simulink model "ConfiguredVirtualVehicleModel"  (R2025b)
settings: Solver=daessc  StartTime=0  StopTime=2474  FixedStep=.001  RelTol=1e-2  EnableMultiTasking=on
StopFcn:
  | %toc
undefined symbols (not defined in the file or in its folder): AccelOvrCmd, CtrlTcuInitGear, DecelOvrCmd, Disabled, DriverPreviewDist, EnblAccelOvr, EnblDecelCmd, EnblSteerCmd, EnvAbsPrs, EnvAirTemp, EnvGrvty, EnvNomFrictionScaling, EnvNominalGrade, EnvWindVelX, EnvWindVelY, EnvWindVelZ, FTP75, MotoFrmInert, MotoFrmLngth, MotoFrmMass, MotoLowrFrntFrkMass, MotoRearArmLngth, MotoRearArmMass, MotoUpprFrntFrkMass, RiderLkAhdPtDstGain, RiderMass, ScnAccTbl, ScnBrkTbl, ScnCRMaxLatAccel, ScnCRRadius, ScnDLCGateLongPos, ScnDLCLatRef, ScnDLCLatRefOffset, ScnDLCLongRefBpt, ScnDLCLongRefStartPos, ScnDLCVehicleWidth, ScnFHCounterDwellTime, ScnFHInitialDwellTime, ScnFHReturnTime, ScnFHRollRateZeroCross, ScnFHSteerAmp, ScnFHSteerSpeed, ScnISHandwheelRate, ScnISMaxHandwheelAng, ScnISMaxLatAccel, ScnISSteerHoldTime, ScnLongPosBpts, ScnLongVelRef, ScnOvalTrackl, ScnOvalTrackpdst, ScnOvalTrackr, ScnSDDwellTime, ScnSDSteerAmp, ScnSDSteerFreq, ScnSSFinalFreq, ScnSSSteerAmp, ScnSSSweepTime, ScnStartTime, ScnStrgAngTbl, ScnStrgTrqTbl ... (+10)
libraries: simulink x16, vehdynlibscenariocommon x9, sm_lib x6, autolibshared x4, nesl_utility x4, vehdynlibviscommon x3, sim3dgroundtruthsensorlib x2, vehdynlibdriver x2, sharedtransform x1, autolibutils x1, sim3dautolib x1, sim3dlib x1
(part 1 of 6)
settings Model: DataDictionary=VirtualMotoTemplate.sldd  ModifiedByFormat=The MathWorks, Inc.  SimulationMode=accelerator  PauseTimes=23.4  PacingRate=0.001000  Creator=The MathWorks, Inc.  LastModifiedBy=The MathWorks, Inc.
settings SolverCC: DaesscMode=Fast  ZeroCrossAlgorithm=Adaptive  AlgebraicLoopSolver=TrustRegion  AutoInsertRateTranBlk=on  InsertRTBMode=Never (minimum delay)  DecoupledContinuousIntegration=on  MinimalZcImpactIntegration=on  MaxZcPerStep=1.0
settings DataIOCC: DSMLogging=off  ReturnWorkspaceOutputs=off
settings OptimizationCC: ReuseModelBlockBuffer=off
settings DebuggingCC: SignalInfNanChecking=error  ArtificialAlgebraicLoopMsg=none  MaskedZcDiagnostic=none  IgnoredZcDiagnostic=none  UnconnectedInputMsg=warning  UnconnectedOutputMsg=warning  UnconnectedLineMsg=warning  PregeneratedLibrarySubsystemCodeDiagnostic=none  SubsystemReferenceDiagnosticForUnitTest=warning  ArithmeticOperatorsInVariantConditions=warning
settings HardwareCC: UseEmbeddedCoderFeatures=off
settings ModelReferenceCC: EnableRefExpFcnMdlSchedulingChecks=on  ModelReferenceMinAlgLoopOccurrences=on  PropagateSignalLabelsOutOfModel=off
settings SFSimCC: SimUseLocalCustomCode=off
settings RTWCC: RTWUseLocalCustomCode=off  GPUComputeCapability=3.5  DLArmComputeVersion=19.05  LargeConstantGeneration=WriteOnlyDNNConstantsToDataFiles
settings ExplorerConfigSet: SimMechanicsOpenEditorOnUpdate=off  InternalSimMechanicsExplorerSettings="<ExplorerConfiguration><canonicalview>default</canonicalview><AnimationSetting><BasePlaybackSpeed>1.0</BasePlaybackSpeed><PlaybackSpeedFactor>0.5</PlaybackSpeedFactor></AnimationSetting><TilePanel><TileInfo><Tiles Columns=\"1\" Count=\"1\" Rows=\"1\"><Column Weight=\"1\"/><Row Weight=\"1\"/><Tile Height=\"1\" Width=\"1\" X=\"0\" Y=\"0\"/></Tiles></TileInfo><SceneInfo><SceneViewer><BGColor><R>0.60000002384185791</R><G>0.60000002384185791</G><B>0.60000002384185791</B></BGColor><Camera><DoPerspective>on</DoPerspective><Position><X>48.3730560002180638</X><Y>0.69720714407681017</Y><Z>1.00624025938607131</Z></Position><Center><X>47.6181790802191784</X><Y>1.35307362107727269</Y><Z>1.00624025938607131</Z></Center><Up><X>0</X><Y>0</Y><Z>1</Z></Up><ViewLimDist>1</ViewLimDist><YLim>0.466307658154998583</YLim><XLim>1.00155607891196818</XLim></Camera></SceneViewer></SceneInfo></TilePanel><MechEditorPanel><Cameras><Camera><Id>Camera1</Id><Value><Name>InplaneRightSide</Name><NativeCamera><PositionTrackingFeature>Motorcycle_Vehicle.Body_Steer_Suspension_Wheels.Body_Steer_Suspension_Wheels.In_Plane_Model.Chassis_Tires_and_Areo.Chassis_Body_Suspension_and_Steering.CHASSIS.Chassis_body.CPRr.Camera.Right.base.R</PositionTrackingFeature><CenterTrackingFeature>Motorcycle_Vehicle.Body_Steer_Suspension_Wheels.Body_Steer_Suspension_Wheels.In_Plane_Model.Chassis_Tires_and_Areo.Chassis_Body_Suspension_and_Steering.CHASSIS.Chassis_body.CPRr.Camera.Right.target.R</CenterTrackingFeature><UpVectorTrackingFeature>Motorcycle_Vehicle.Body_Steer_Suspension_Wheels.Body_Steer_Suspension_Wheels.In_Plane_Model.Chassis_Tires_and_Areo.Chassis_Body_Suspension_and_Steering.CHASSIS.Chassis_body.CPRr.Camera.Right.target.R</UpVectorTrackingFeature><CenterTrackingOrigin>off</CenterTrackingOrigin><CenterTrackingDirection>-Y</CenterTrackingDirection><UpVectorTrackingDirection>-Z</UpVectorTrackingDirection></NativeCamera></Value></Camera><Camera><Id>Camera2</Id><Value><Name>OutofPlaneRightSide</Name><NativeCamera><PositionTrackingFeature>Motorcycle_Vehicle.Body_Steer_Suspension_Wheels.Body_Steer_Suspension_Wheels.Out_of_Plane_Model.Chassis_Tires_and_Areo.Chassis_Body_Suspension_and_Steering.CHASSIS.Chassis_body.CPRr.Camera.Right.base.R</PositionTrackingFeature><CenterTrackingFeature>Motorcycle_Vehicle.Body_Steer_Suspension_Wheels.Body_Steer_Suspension_Wheels.Out_of_Plane_Model.Chassis_Tires_and_Areo.Chassis_Body_Suspension_and_Steering.CHASSIS.Chassis_body.CPRr.Camera.Right.base.R</CenterTrackingFeature><UpVectorTrackingFeature>Motorcycle_Vehicle.Body_Steer_Suspension_Wheels.Body_Steer_Suspension_Wheels.Out_of_Plane_Model.Chassis_Tires_and_Areo.Chassis_Body_Suspension_and_Steering.CHASSIS.Chassis_body.CPRr.Camera.Right.base.R</UpVectorTrackingFeature><CenterTrackingOrigin>off</CenterTrackingOrigin><CenterTrackingDirection>-Y</CenterTrackingDirection><UpVectorTrackingDirection>-Z</UpVectorTrackingDirection></NativeCamera></Value></Camera></Cameras><GfxPanelCameraMap><MapElement CameraMLId=\"Camera2\" GfxPanelIndex=\"0\"/></GfxPanelCameraMap><VideoCreator><PlaybackSpeedRatio>1.0</PlaybackSpeedRatio><FrameRate>30</FrameRate><VideoFormat>Motion JPEG AVI</VideoFormat><FrameSize>auto</FrameSize></VideoCreator></MechEditorPanel></ExplorerConfiguration>"

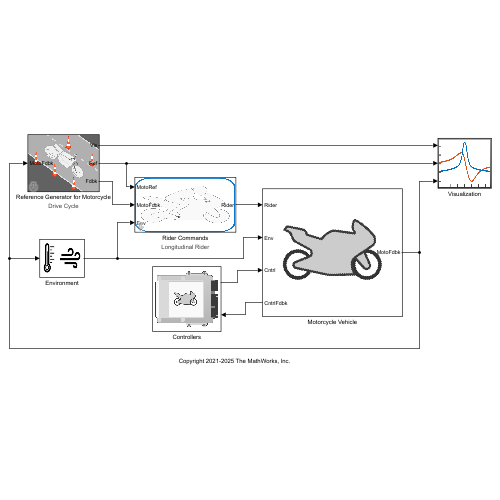
[thumbnail: Simulink's stored preview of the top-level diagram]
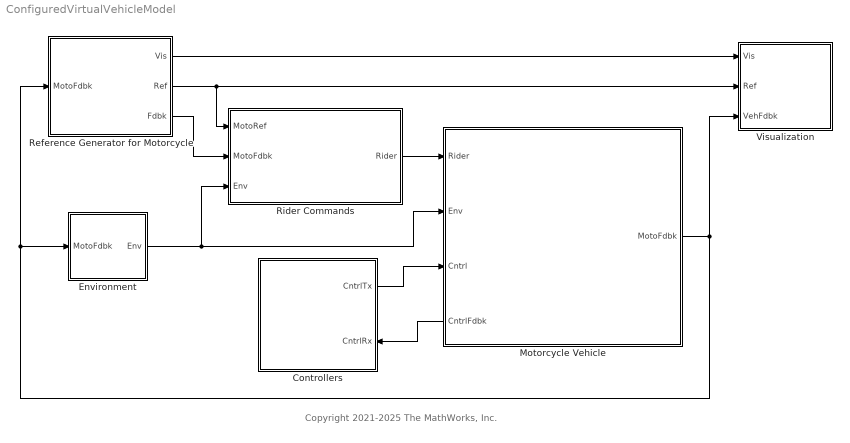
== system ConfiguredVirtualVehicleModel ==
  note: Copyright 2021-2025 The MathWorks, Inc.
  Controllers : Subsystem
      settings: PortSchema="{\"entries\":[{\"content\":{\"sides\":[{\"content\":{},\"type\":\"ConnectorPlacement.EquallySpacedRectSide\",\"uuid\":\"d3abfdf3-59f3-4762-8e4e-957745a11e2c\"},{\"content\":{\"connectorIds\":[\"Out1\",\"In1\"],\"side\":\"RIGHT\"},\"type\":\"ConnectorPlacement.EquallySpacedRectSide\",\"uuid\":\"4c115717-9c17-4631-bd95-1f831e7f83d7\"},{\"content\":{\"side\":\"TOP\"},\"type\":\"ConnectorPlacement.EquallySpacedRectSide\",\"uuid\":\"d2ccb451-5fc1-4147-9a0c-1582624fa182\"}]},\"type\":\"ConnectorPlacement.EquallySpacedConnector\",\"uuid\":\"cab9e2c1-ce8a-4f9c-a024-cef64f8d49c6\"}],\"packageUris\":[\"http://schema.mathworks.com/mf0/Connector/R2020b\"],\"version\":\"1.0\"}"
      mask Display: image('motoECU.png')
  Environment : Subsystem
      mask Display: image('Enviroment.png')
  Motorcycle Vehicle : Subsystem
      settings: PortSchema="{\"entries\":[{\"content\":{\"sides\":[{\"content\":{\"connectorIds\":[\"In1\",\"In2\",\"In3\",\"Out2\"]},\"type\":\"ConnectorPlacement.EquallySpacedRectSide\",\"uuid\":\"175d7041-2aff-4cd5-b9c0-3998d48105ea\"},{\"content\":{\"connectorIds\":[\"Out1\"],\"side\":\"RIGHT\"},\"type\":\"ConnectorPlacement.EquallySpacedRectSide\",\"uuid\":\"0f698ea4-f06f-4552-98b1-af1f0960853e\"},{\"content\":{\"side\":\"TOP\"},\"type\":\"ConnectorPlacement.EquallySpacedRectSide\",\"uuid\":\"8127d405-6a03-4548-a956-3e3bb7246319\"}]},\"type\":\"ConnectorPlacement.EquallySpacedConnector\",\"uuid\":\"b217a386-2802-4b5f-8626-423e606b91b2\"}],\"packageUris\":[\"http://schema.mathworks.com/mf0/Connector/R2020b\"],\"version\":\"1.0\"}"
      mask Display: image('moto.png')
  Reference Generator for Motorcycle : Subsystem  Priority=1  mask(Reference Generator){manType=Drive Cycle, manOverride=off, SpdCtrlOverride=off, prevType=Drive Cycle, t_start=ScnStartTime, xdot_r=ScnLongVelRef, xdotUnit=mph, steerDir=off, aMode=2, RidTrajContGl=RiderLkAhdPtDstGain, omega_hw=ScnISHandwheelRate, theta_max=ScnISMaxHandwheelAng, t_stop=ScnISSteerHoldTime, ay_max=ScnISMaxLatAccel, ay_stop=off, XGate=ScnDLCGateLongPos, xStart=ScnDLCLongRefStartPos, vehW=ScnDLCVehicleWidth, latoff=ScnDLCLatRefOffset, latRefbp=ScnDLCLongRefBpt, latRef=ScnDLCLatRef, t_sweep=ScnSSSweepTime, theta_hw=ScnSSSteerAmp, theta_hw_final=ScnSSFinalFreq, steerF=ScnSDSteerFreq, steerA=ScnSDSteerAmp, tdwell=ScnSDDwellTime, R=ScnCRRadius*0.5, cr_ay_max=ScnCRMaxLatAccel, cr_ay_stop=off, Trajl=ScnOvalTrackl, Trajr=ScnOvalTrackr, Trajpointdist=ScnOvalTrackpdst, TrajDataSource=Variable, TrajDatFileCSV=ScnUDTrackCSVFile, TrajDatFile=ScnUDTrackMATFile, CoordinateX=ScnUDTrackCoordX, CoordinateY=ScnUDTrackCoordY, steerRate=ScnFHSteerSpeed, steerAFH=ScnFHSteerAmp, pFdbk=off, tDwell1=ScnFHInitialDwellTime, tDwell2=ScnFHCounterDwellTime, tSteer3=ScnFHReturnTime, pZero=ScnFHRollRateZeroCross, cycleVar=FTP75, xdot_wot1=90, srcUnit=mph, t_wot2=ScnTimeToStrtDecel, OverrideType=Steering torque override, ActType=Time-based activation, TimeBpts=ScnTimeBpts, LongPosBpts=ScnLongPosBpts, StrgAngTbl=ScnStrgAngTbl, StrgTrqTbl=ScnStrgTrqTbl, AccTbl=ScnAccTbl, BrkTbl=ScnBrkTbl, simTime=2474, engine3D=Disabled, SceneDesc=Open surface, dt3D=.03, defaultPos=User-specified, X_o=0, Y_o=0, Z_o=0, phi_o=0, theta_o=0, psi_o=0}
      mask prompts: manType "vdynblks:vehdynManConstantRadius:blkPrm_manType"; manOverride "vdynblks:vehdynManConstantRadius:blkPrm_manOverride"; SpdCtrlOverride "Speed control override"; t_start "vdynblks:vehdynManConstantRadius:blkPrm_t_start"; xdot_r "vdynblks:vehdynManConstantRadius:blkPrm_xdot_r"; xdotUnit "Simulink:blkprm_prompts:OutputUnit_EditField"; steerDir "vdynblks:vehdynManConstantRadius:blkPrm_steerDir"; RidTrajContGl "Gain that determines the distance to the look ahead point, RidContGl [s]:"; omega_hw "vdynblks:vehdynManConstantRadius:blkPrm_omega_hw"; theta_max "vdynblks:vehdynManConstantRadius:blkPrm_theta_max"; t_stop "vdynblks:vehdynManConstantRadius:blkPrm_t_stop"; ay_max "vdynblks:vehdynManConstantRadius:blkPrm_ay_max"; ay_stop "vdynblks:vehdynManConstantRadius:blkPrm_ay_stop"; XGate "vdynblks:vehdynManConstantRadius:blkPrm_XGate"; xStart "vdynblks:vehdynManConstantRadius:blkPrm_xStart"; vehW "vdynblks:vehdynManConstantRadius:blkPrm_vehW"; latoff "vdynblks:vehdynManConstantRadius:blkPrm_latoff"; latRefbp "vdynblks:vehdynManConstantRadius:blkPrm_latRefbp"; latRef "vdynblks:vehdynManConstantRadius:blkPrm_latRef"; t_sweep "vdynblks:vehdynManConstantRadius:blkPrm_t_sweep"; theta_hw "vdynblks:vehdynManConstantRadius:blkPrm_theta_hw"; theta_hw_final "vdynblks:vehdynManConstantRadius:blkPrm_theta_hw_final"; steerF "vdynblks:vehdynManConstantRadius:blkPrm_steerF"; steerA "vdynblks:vehdynManConstantRadius:blkPrm_steerA"; tdwell "vdynblks:vehdynManConstantRadius:blkPrm_tdwell"; R "vdynblks:vehdynManConstantRadius:blkPrm_R"; cr_ay_max "vdynblks:vehdynManConstantRadius:blkPrm_cr_ay_max"; cr_ay_stop "vdynblks:vehdynManConstantRadius:blkPrm_cr_ay_stop"; Trajl "vdynblks:vehdynManOvalTrack:blkDlg_OTStLen"; Trajr "vdynblks:vehdynManOvalTrack:blkDlg_OTTRad"; Trajpointdist "vdynblks:vehdynManOvalTrack:blkDlg_OTCIntvl"; TrajDataSource "vdynblks:vehdynManUserDefinedTrack:blkDlg_DatSrcGroup"; TrajDatFileCSV "vdynblks:vehdynManUserDefinedTrack:blkDlg_TrkDatFile"; TrajDatFile "vdynblks:vehdynManUserDefinedTrack:blkDlg_TrkDatFile"; CoordinateX "vdynblks:vehdynManUserDefinedTrack:blkDlg_UDTVarX"; CoordinateY "vdynblks:vehdynManUserDefinedTrack:blkDlg_UDTVarY"; steerRate "vdynblks:vehdynManFishook:blkPrm_steerRate"; steerAFH "vdynblks:vehdynManConstantRadius:blkPrm_steerAFH"; pFdbk "vdynblks:vehdynManFishook:blkPrm_pFdbk"; tDwell1 "vdynblks:vehdynManFishook:blkPrm_tDwell1"; tDwell2 "vdynblks:vehdynManFishook:blkPrm_tDwell2"; tSteer3 "vdynblks:vehdynManFishook:blkPrm_tSteer3"; pZero "vdynblks:vehdynManFishook:blkPrm_pZero"; cycleVar "autoblks_shared:autoblkDriveCycleSource:blkPrm_cycleVar"; xdot_wot1 "autoblks_shared:autoblkDriveCycleSource:blkPrm_xdot_wot1"; srcUnit "autoblks_shared:autoblkDriveCycleSource:blkPrm_srcUnit"; t_wot2 "autoblks_shared:autoblkDriveCycleSource:blkPrm_t_wot2"; OverrideType "Override type:"; ActType "Test activation type:"; TimeBpts "Time breakpoints, TimeBpts [t]:"; LongPosBpts "Longitudinal position breakpoints, LongPosBpts [m]:"; StrgAngTbl "Steering angle table, StrgAngTbl [rad]:"; StrgTrqTbl "Steering torque table, StrgTrqTbl [N*m]:"; AccTbl "Acceleration table, AccTbl [-]:"; BrkTbl "Brake table, BrkTbl [-]:"; simTime "vdynblks:vehdynManConstantRadius:blkPrm_simTime"; engine3D "vdynblks:vehdynManConstantRadius:blkPrm_engine3D"; SceneDesc "vdynblks:vehdynManConstantRadius:blkPrm_SceneDesc"; dt3D "vdynblks:vehdynManConstantRadius:blkPrm_dt3D"; X_o "vdynblks:vehdynManConstantRadius:blkPrm_X_o"; Y_o "vdynblks:vehdynManConstantRadius:blkPrm_Y_o"; Z_o "vdynblks:vehdynManConstantRadius:blkPrm_Z_o"; phi_o "vdynblks:vehdynManConstantRadius:blkPrm_phi_o"; theta_o "vdynblks:vehdynManConstantRadius:blkPrm_theta_o"; psi_o "vdynblks:vehdynManConstantRadius:blkPrm_psi_o"
      mask help: vdynblks:vehdynManConstantRadius:blkDesc
      mask init:
      | [~]=vdynblksrefconfig(gcb,0);
      settings: AttributesFormatString=%<manType>
      mask Help: eval('vdynblkshelp(''vdmtrrefgen'')');
      mask TypeOptions manType: vdynblks:vehdynManUserDefinedTrack:blkDlg_DC | vdynblks:vehdynManUserDefinedTrack:blkDlg_MMD
      mask Callback manType: [~]=vdynblksrefconfig(gcb,1);
      mask Callback manOverride: [~]=vdynblksrefconfig(gcb,3);
      mask Callback SpdCtrlOverride: [~] = vdynblksrefconfig(gcb,5);
      mask TypeOptions prevType: Double Lane Change | Increasing Steer | Swept Sine | Sine with Dwell | Constant Radius | Fishhook | Drive Cycle | Manual Maneuver Design | Constant Radius RCP | vdynblks:vehdynManOvalTrack:blkDlg_OTGroup | vdynblks:vehdynManUserDefinedTrack:blkDlg_UDTGroup
      mask TypeOptions xdotUnit: Reference Generator/Longitudinal Maneuver Tracking/refUnit/Unit | Reference Generator/Constant Radius/xdotUnit | Reference Generator/Double Lane Change/Double Lane Change/xdotUnit | Reference Generator/Drive Cycle/Drive Cycle Source/outUnit | Reference Generator/Fishhook/Fishhook/xdotUnit | Reference Generator/Increasing Steer/Increasing Steer/xdotUnit | Reference Generator/Sine with Dwell/Sine With Dwell/xdotUnit | Reference Generator/Swept Sine/Swept Sine/xdotUnit
      mask TypeOptions steerDir: Reference Generator/Sine with Dwell/Sine With Dwell/steerDir | Reference Generator/Fishhook/Fishhook/steerDir | Reference Generator/Constant Radius/steerDir | Reference Generator/Increasing Steer/Increasing Steer/steerDir
      mask TypeOptions omega_hw: Reference Generator/Increasing Steer/Increasing Steer/omega_hw
      mask TypeOptions theta_max: Reference Generator/Increasing Steer/Increasing Steer/theta_max
      mask TypeOptions t_stop: Reference Generator/Increasing Steer/Increasing Steer/t_stop
      mask TypeOptions ay_max: Reference Generator/Increasing Steer/Increasing Steer/ay_max
      mask TypeOptions ay_stop: Reference Generator/Increasing Steer/Increasing Steer/ay_stop
      mask Callback ay_stop: [~] = vdynblksrefconfig(gcb,10);
      mask TypeOptions XGate: Reference Generator/Double Lane Change/Double Lane Change/XGate
      mask TypeOptions xStart: Reference Generator/Double Lane Change/Double Lane Change/xStart
      mask TypeOptions vehW: Reference Generator/Double Lane Change/Double Lane Change/vehW
      mask TypeOptions latoff: Reference Generator/Double Lane Change/Double Lane Change/latoff
      mask TypeOptions latRefbp: Reference Generator/Double Lane Change/Double Lane Change/latRefbp
      mask TypeOptions latRef: Reference Generator/Double Lane Change/Double Lane Change/latRef
      mask TypeOptions t_sweep: Reference Generator/Swept Sine/Swept Sine/t_sweep
      mask TypeOptions theta_hw: Reference Generator/Swept Sine/Swept Sine/theta_hw
      mask TypeOptions theta_hw_final: Reference Generator/Swept Sine/Swept Sine/theta_hw_final
      mask TypeOptions steerF: Reference Generator/Sine with Dwell/Sine With Dwell/steerF
      mask TypeOptions steerA: Reference Generator/Sine with Dwell/Sine With Dwell/steerA
      mask TypeOptions tdwell: Reference Generator/Sine with Dwell/Sine With Dwell/tdwell
      mask TypeOptions R: Reference Generator/Constant Radius/R
      mask TypeOptions cr_ay_max: Reference Generator/Constant Radius/ay_max
      mask TypeOptions cr_ay_stop: Reference Generator/Constant Radius/ay_stop
      mask Callback cr_ay_stop: [~] = vdynblksrefconfig(gcb,11);
      mask TypeOptions Trajl: Reference Generator/Moto Target Trajectory/Trajl
      mask TypeOptions Trajr: Reference Generator/Moto Target Trajectory/Trajr
      mask TypeOptions Trajpointdist: Reference Generator/Moto Target Trajectory/Trajpointdist
      mask TypeOptions TrajDataSource: Reference Generator/Moto Target Trajectory/TrajDataSource
      mask Callback TrajDataSource: [~]=vdynblksrefconfig(gcb,6);
      mask TypeOptions TrajDatFileCSV: Reference Generator/Moto Target Trajectory/TrajDatFileCSV
      mask TypeOptions TrajDatFile: Reference Generator/Moto Target Trajectory/TrajDatFile
      mask TypeOptions CoordinateX: Reference Generator/Moto Target Trajectory/CoordinateX
      mask TypeOptions CoordinateY: Reference Generator/Moto Target Trajectory/CoordinateY
      mask TypeOptions steerRate: Reference Generator/Fishhook/Fishhook/steerRate
      mask TypeOptions pFdbk: Reference Generator/Fishhook/Fishhook/pFdbk
      mask Callback pFdbk: [~]=vdynblksrefconfig(gcb,12);
      mask TypeOptions tDwell1: Reference Generator/Fishhook/Fishhook/tDwell1
      mask TypeOptions tDwell2: Reference Generator/Fishhook/Fishhook/tDwell2
      mask TypeOptions tSteer3: Reference Generator/Fishhook/Fishhook/tSteer3
      mask TypeOptions pZero: Reference Generator/Fishhook/Fishhook/pZero
      mask TypeOptions cycleVar: Reference Generator/Drive Cycle/Drive Cycle Source/cycleVar
      mask Callback cycleVar: [~]=vdynblksrefconfig(gcb,13);
      mask TypeOptions xdot_wot1: Reference Generator/WOT/Drive Cycle Source/xdot_wot1
      mask TypeOptions srcUnit: Reference Generator/WOT/Drive Cycle Source/srcUnit
      mask TypeOptions t_wot2: Reference Generator/WOT/Drive Cycle Source/t_wot2
      mask TypeOptions OverrideType: Steering torque override | Steering angle override
      mask Callback OverrideType: [~]=vdynblksrefconfig(gcb,8);
      mask TypeOptions ActType: Time-based activation | Logitudinal position-based activation
      mask Callback ActType: [~]=vdynblksrefconfig(gcb,9);
      mask TypeOptions engine3D: 3D Engine/engine3D
      mask Callback engine3D: [~]=vdynblksrefconfig(gcb,4);
      mask TypeOptions SceneDesc: 3D Engine/SceneDesc
      mask Callback SceneDesc: [~] = vdynblks3Dsceneconfig(gcb);
      mask TypeOptions dt3D: 3D Engine/dt3D
      mask TypeOptions defaultPos: Recommended for scene | User-specified
      mask Callback defaultPos: [~] = vdynblksmdlWSconfig(gcb,false);
      mask TypeOptions X_o: 3D Engine/X_o | Reference Generator/Double Lane Change/Double Lane Change/X_o | Reference Generator/Constant Radius/X_o
      mask TypeOptions Y_o: 3D Engine/Y_o | Reference Generator/Double Lane Change/Double Lane Change/Y_o | Reference Generator/Constant Radius/Y_o
      mask TypeOptions Z_o: 3D Engine/Z_o
      mask TypeOptions phi_o: 3D Engine/phi_o | Reference Generator/Double Lane Change/Double Lane Change/psi_o
      mask TypeOptions theta_o: 3D Engine/theta_o
      mask TypeOptions psi_o: 3D Engine/psi_o
      mask DialogControl modTab Prompt: vdynblks:vehdynManConstantRadius:blkDlg_modTab
      mask DialogControl configGroup Prompt: vdynblks:vehdynManConstantRadius:blkDlg_configGroup
      mask DialogControl manType Prompt: Maneuver:
      mask DialogControl manOverride Prompt: Use maneuver-specific driver, initial position, and scene
      mask DialogControl t_start Prompt: Maneuver start time, t_start [s]:
      mask DialogControl xdot_r Prompt: Longitudinal velocity reference, xdot_r:
      mask DialogControl xdotUnit Prompt: Unit (e.g., m, m/s^2, N*m):
      mask DialogControl steerDir Prompt: Maneuver direction, steerDir:
      mask DialogControl ISGroup Prompt: vdynblks:vehdynManConstantRadius:blkDlg_ISGroup
      mask DialogControl omega_hw Prompt: Handwheel rate, omega_hw [deg/s]:
      mask DialogControl theta_max Prompt: Maximum handwheel angle, theta_max [deg]:
      mask DialogControl t_stop Prompt: Steering hold time after max angle reached, t_stop [s]:
      mask DialogControl ay_max Prompt: Lateral acceleration threshold, ay_max [g]:
      mask DialogControl ay_stop Prompt: Stop simulation at lateral acceleration threshold:
      mask DialogControl DLCGroup Prompt: vdynblks:vehdynManConstantRadius:blkDlg_DLCGroup
      mask DialogControl XGate Prompt: Inertial longitudinal position of gate entrance, XGate [m]:
      mask DialogControl xStart Prompt: Distance after target velocity to begin reference, xStart [m]:
      mask DialogControl vehW Prompt: Distance between inside and outside cone boundaries, vehW [m]:
      mask DialogControl latoff Prompt: Lateral offset, latoff [m]:
      mask DialogControl latRefbp Prompt: Lateral reference position breakpoints [m]:
      mask DialogControl latRef Prompt: Lateral reference data, latRef [m]:
      mask DialogControl SSGroup Prompt: vdynblks:vehdynManConstantRadius:blkDlg_SSGroup
      mask DialogControl t_sweep Prompt: Swept time, t_sweep [s]:
      mask DialogControl theta_hw Prompt: Steering amplitude, theta_hw [deg]:
      mask DialogControl theta_hw_final Prompt: Final frequency, theta_hw_final [Hz]:
      mask DialogControl SDGroup Prompt: vdynblks:vehdynManConstantRadius:blkDlg_SDGroup
      mask DialogControl steerF Prompt: Steer frequency, steerF [Hz]:
      mask DialogControl steerA Prompt: Steer amplitude, steerA [deg]:
      mask DialogControl tdwell Prompt: Dwell time, tdwell [s]:
      mask DialogControl CRGroup Prompt: vdynblks:vehdynManConstantRadius:blkDlg_CRGroup
      mask DialogControl R Prompt: Radius value, R [m]:
      mask DialogControl cr_ay_max Prompt: Lateral acceleration threshold, cr_ay_max [g]:
      mask DialogControl cr_ay_stop Prompt: Stop simulation at lateral acceleration threshold
      mask DialogControl TPOvalGroup Prompt: vdynblks:vehdynManOvalTrack:blkDlg_OTGroup
      mask DialogControl Trajl Prompt: Straight Segment Length, traj_l [m]:
      mask DialogControl Trajr Prompt: Turn Radius, traj_r [m]:
      mask DialogControl Trajpointdist Prompt: Coordinate Interval, trajp_dist [m]:
      mask DialogControl OvalTrajConfBtn Prompt: vdynblks:vehdynManOvalTrack:blkDlg_PlotBtn
      mask DialogControl OvalTrajConfBtn Callback: [~]=vdynblksrefconfig(gcb,7);
      mask DialogControl TPUserDefGroup Prompt: vdynblks:vehdynManUserDefinedTrack:blkDlg_UDTGroup
      mask DialogControl TrajDataSource Prompt: Data Source:
      mask DialogControl TrajDatFileCSV Prompt: Track Data File:
      mask DialogControl TrajDatFile Prompt: Track Data File:
      mask DialogControl CoordinateX Prompt: Inertial X-axis Coordinate, udt_coord_x [m]:
      mask DialogControl CoordinateY Prompt: Inertial Y-axis Coordinate, udt_coord_y [m]:
      mask DialogControl UserDefinedTrajConfBtn Prompt: vdynblks:vehdynManUserDefinedTrack:blkDlg_PlotBtn
      mask DialogControl UserDefinedTrajConfBtn Callback: [~]=vdynblksrefconfig(gcb,7);
      mask DialogControl FHGroup Prompt: vdynblks:vehdynManConstantRadius:blkDlg_FHGroup
      mask DialogControl steerRate Prompt: Steer and countersteer speed, steerRate [deg/s]:
      mask DialogControl steerAFH Prompt: Steer amplitude, steerAFH, [deg]:
      mask DialogControl pFdbk Prompt: Use roll rate to determine initial steer dwell time
      mask DialogControl tDwell1 Prompt: Initial dwell time, tDwell1 [s]:
      mask DialogControl tDwell2 Prompt: Countersteer dwell time, tDwell2 [s]:
      mask DialogControl tSteer3 Prompt: Return to center time, tSteer3 [s]:
      mask DialogControl pZero Prompt: Roll rate countersteer initiation zero crossing threshold, pZero [deg/s]:
      mask DialogControl pZero Tooltip: vdynblks:vehdynManFishook:blkDlg_pZeroToolTip
      mask DialogControl DCGroup Prompt: Drive Cycle
      mask DialogControl cycleVar Prompt: Drive cycle source:
      mask DialogControl openDCbutton Prompt: Click for all configuration options
      mask DialogControl openDCbutton Callback:
      | [~]=vdynblksrefconfig(gcb,0);
      | aMaskObj = Simulink.Mask.get(gcb);
      | aDlgHdl = aMaskObj.getDialogHandle();
      | aDlgHdl.apply;
      | cycleVar = get_param(gcb,'cycleVar');
      | if strcmp(cycleVar,'Wide Open Throttle (WOT)')
      |     open_system([gcb '/Reference Generator/WOT/Drive Cycle Source'],"mask")
      | else
      | open_system([gcb '/Reference Generator/Drive Cycle/Drive Cycle Source'],"mask")
      | end
      mask DialogControl xdot_wot1 Prompt: Nominal reference speed, xdot_wot1 []:
      mask DialogControl srcUnit Prompt: Source velocity units (e.g., m/s, km/h, mph):
      mask DialogControl t_wot2 Prompt: Time to start deceleration, t_wot2 [s]:
      mask DialogControl MOGroup Prompt: Manual Maneuver Design
      mask DialogControl simTime Prompt: Simulation time, simTime [s]:
      mask DialogControl simUpdate Prompt: vdynblks:vehdynManConstantRadius:blkDlg_simUpdate
      mask DialogControl simUpdate Callback: [~]=vdynblksrefconfig(gcb,2);
      mask DialogControl sim3DTab Prompt: vdynblks:vehdynManConstantRadius:blkDlg_sim3DTab
      mask DialogControl sim3DGroup Prompt: vdynblks:vehdynManConstantRadius:blkDlg_sim3DGroup
      mask DialogControl engine3D Prompt: 3D Engine:
      mask DialogControl SceneDesc Prompt: Scene:
      mask DialogControl dt3D Prompt: 3D Engine frame rate, dt3D [s]:
      mask DialogControl posSetupDesc Prompt: To use these initial vehicle positions, first Apply the initial values and then click Update the model workspaces with the initial values.
      mask DialogControl X_o Prompt: Initial longitudinal position, X_o [m]:
      mask DialogControl Y_o Prompt: Initial lateral position, Y_o [m]:
      mask DialogControl Z_o Prompt: Initial vertical position, Z_o [m]:
      mask DialogControl phi_o Prompt: Initial roll angle, phi_o [rad]:
      mask DialogControl theta_o Prompt: Initial pitch angle, theta_o [rad]:
      mask DialogControl psi_o Prompt: Initial yaw angle, psi_o [rad]:
      mask Display: image('$imagefile'); % Use "Edit Image" on toolstrip to change.
  Rider Commands : Subsystem  VariantControl=0  mask{driverType=Longitudinal Rider, TorqueControlType=No torque control, A=0, D=0.1, I=5, P=150, OutSatLowLmt=-100, OutSatUpLmt=100}
      mask prompts: driverType "Rider type"; TorqueControlType "Torque control"; A "vdynblks:vehdynSteeringSystem:blkPrm_AntiwindGain"; D "vdynblks:vehdynSteeringSystem:blkPrm_DGain"; I "vdynblks:vehdynSteeringSystem:blkPrm_IGain"; P "vdynblks:vehdynSteeringSystem:blkPrm_PGain"; OutSatLowLmt "vdynblks:vehdynSteeringSystem:blkPrm_OutSatLowLmt"; OutSatUpLmt "vdynblks:vehdynSteeringSystem:blkPrm_OutSatUpLmt"
      mask init:
      | [~]=vdynblksdrvrconfig(gcb);
      settings: AttributesFormatString=%<driverType>
      mask Help: eval('vdynblkshelp(''vdmtrrider'')');
      mask TypeOptions driverType: Longitudinal Rider | Open Loop
      mask Callback driverType: [~]=vdynblksdrvrconfig(gcb);
      mask TypeOptions TorqueControlType: Torque PID control | No torque control | Look ahead point model | PID Control
      mask DialogControl A Prompt: Integral anti-windup gain, A []:
      mask DialogControl D Prompt: Derivative gain, D []:
      mask DialogControl I Prompt: Integral gain, I []:
      mask DialogControl P Prompt: Proportional gain, P []:
      mask DialogControl OutSatLowLmt Prompt: Steering torque output saturation lower limit, OutSatLowLmt [Nm]:
      mask DialogControl OutSatUpLmt Prompt: Steering torque output saturation upper limit, OutSatUpLmt [Nm]:
      mask Display: image('rider.png'); % Use "Edit Image" on toolstrip to change.
  Visualization : Subsystem
      mask Display: image('Visualization.png')
  wires:
  Controllers/1(CntrlTx) -> Motorcycle Vehicle/3(Cntrl)
  Motorcycle Vehicle/2(CntrlFdbk) -> Controllers/1(CntrlRx)
  Reference Generator for Motorcycle/2(" Ref") -> Visualization/2(Ref), Rider Commands/1(MotoRef)
  Reference Generator for Motorcycle/3(" Fdbk") -> Rider Commands/2(MotoFdbk)
  Environment/1(Env) -> Rider Commands/3(Env), Motorcycle Vehicle/2(Env)
  Motorcycle Vehicle/1(MotoFdbk) -> Reference Generator for Motorcycle/1("MotoFdbk "), Environment/1(MotoFdbk), Visualization/3(VehFdbk)
  Rider Commands/1(Rider) -> Motorcycle Vehicle/1(Rider)
  Reference Generator for Motorcycle/1(" Vis") -> Visualization/1(Vis)

== system ConfiguredVirtualVehicleModel/Controllers ==
  CntrlRx : Inport
  Battery Management System (BMS) : Subsystem  Variant=on  VariantControlMode=label  LabelModeActiveChoice=NoBMS
  Brake Control Unit (BCU) : Subsystem  Variant=on  VariantChoicesSpecifier={'OpenLoopController'}  VariantControlMode=label  LabelModeActiveChoice=OpenLoopController
  Bus Creator : BusCreator  Inputs=1
  Bus Creator1 : BusCreator  Inputs=1
  Bus Creator3 : BusCreator  Inputs=3
  Bus Creator4 : BusCreator  Inputs=2
  Bus Selector3 : BusSelector  OutputSignals=Battery.BMSSensors
  Engine Control Unit (ECU) : Subsystem  Variant=on  VariantChoicesSpecifier={'MotoSimpleECU'}  VariantControlMode=label  LabelModeActiveChoice=MotoSimpleECU
  Subsystem : Subsystem
  Subsystem1 : Subsystem
  Subsystem2 : Subsystem
  Subsystem3 : Subsystem
  Subsystem4 : Subsystem
  Transmission Control Unit (TCU) : Subsystem  Variant=on  VariantChoicesSpecifier={'RiderPassThrough'}  VariantControlMode=label  VariantControl=Variant1  LabelModeActiveChoice=RiderPassThrough
  Vehicle Control Unit (VCU) : Subsystem  Variant=on  VariantChoicesSpecifier={'NoVCU'}  VariantControlMode=label  LabelModeActiveChoice=NoVCU
  BusElementOut : Outport  PortName=CntrlTx  Element=BMS
  BusElementOut1 : Outport  PortName=CntrlTx  Element=Brake
  BusElementOut2 : Outport  PortName=CntrlTx  Element=Transmission
  BusElementOut3 : Outport  PortName=CntrlTx  Element=ECU
  BusElementOut4 : Outport  PortName=CntrlTx  Element=VCU
  wires:
  Bus Creator/1 -> BusElementOut3/1  "ECU"
  Bus Creator1/1 -> BusElementOut2/1  "Transmission"
  Engine Control Unit (ECU)/1(EngTrqCmd) -> Bus Creator/1  "EngTrqCmd"
  Transmission Control Unit (TCU)/1(" Gear") -> Bus Creator1/1  "GearCmd"
  CntrlRx/1 -> Subsystem3/1(CntrlRx), Bus Selector3/1, Subsystem2/2(CntrlRx), Subsystem1/2(CntrlRx), Subsystem/3(Cntrl)
  Bus Selector3/1 -> Battery Management System (BMS)/1(BMSSensors)  "<BMSSensors>"
  Battery Management System (BMS)/2(BMSCmd) -> Bus Creator4/2  "BMSCmd"
  Bus Creator4/1 -> [BMS], BusElementOut/1  "BMS"
  Battery Management System (BMS)/1(BMSInfo) -> Bus Creator4/1  "BMSInfo"
  Bus Creator3/1 -> [VCU], BusElementOut4/1  "VCU"
  Vehicle Control Unit (VCU)/1(EngTrqCmd) -> Bus Creator3/1  "EngTrqCmd"
  Vehicle Control Unit (VCU)/2(EMTrqCmd) -> Bus Creator3/2  "EMTrqCmd"
  Vehicle Control Unit (VCU)/3(VcuBrkPrsCmd) -> Bus Creator3/3  "VcuBrkPrsCmd"
  [Brake] -> Subsystem/1(Brake)
  [BMS] -> Subsystem/2(BMS)
  Subsystem/1(<AccFdbk>) -> Vehicle Control Unit (VCU)/1(AccelPdl)
  Subsystem/2(<MotoXVel>) -> Vehicle Control Unit (VCU)/2(VehSpdFdbk)
  Subsystem/3(<BattSoc>) -> Vehicle Control Unit (VCU)/3(BattSoc)
  Subsystem/4(<EMSpd>) -> Vehicle Control Unit (VCU)/4(EMSpd)
  Subsystem/5(<PackVoltage>) -> Vehicle Control Unit (VCU)/5(BattPackVolt)
  Subsystem/6(<pqr>) -> Vehicle Control Unit (VCU)/6(pqr)
  Subsystem/7(<SteerFdbk>) -> Vehicle Control Unit (VCU)/7(SteerCmd)
  Subsystem/8(<thetasteer>) -> Vehicle Control Unit (VCU)/8(SteerWhlAng)
  Subsystem/9(<Gear>) -> Vehicle Control Unit (VCU)/9(TransGear)
  Subsystem/10(<BrkPrsCmd>) -> Vehicle Control Unit (VCU)/10(BcuBrkPrsCmd)
  Subsystem/11(<SOC_CC>) -> Vehicle Control Unit (VCU)/11(BMSSOC)
  Subsystem/12(<DischargeCurrentLimit>) -> Vehicle Control Unit (VCU)/12(BMSDischrgCurrLmt)
  Subsystem/13(<ChargeCurrentLimit>) -> Vehicle Control Unit (VCU)/13(BMSChrgCurrLmt)
  [VCU] -> Subsystem1/1(VCU)
  [Brake] -> Subsystem1/3(Brake)
  Subsystem1/1(<EngTrqCmd>) -> Engine Control Unit (ECU)/1(TrqCmd)
  Subsystem1/2(<EngSpd>) -> Engine Control Unit (ECU)/2(EngSpd)
  Subsystem1/3(<ABSFlag>) -> Engine Control Unit (ECU)/3(ABSFlag)
  [Brake] -> Subsystem2/1(Brake)
  Subsystem2/1(<ABSFlag>) -> Transmission Control Unit (TCU)/1(ABSFlag)
  Subsystem2/2(<AccFdbk>) -> Transmission Control Unit (TCU)/2(Accel)
  Subsystem2/3(<DecelFdbk>) -> Transmission Control Unit (TCU)/3(BrkCmd)
  Subsystem2/4(<GearFdbk>) -> Transmission Control Unit (TCU)/4(GearReq)
  Subsystem2/5(<EngSpd>) -> Transmission Control Unit (TCU)/5(EngSpd)
  Subsystem2/6(<Omega>) -> Transmission Control Unit (TCU)/6(Omega)
  Subsystem3/1(<DecelFdbk>) -> Brake Control Unit (BCU)/1(DecelFdbk)
  Subsystem3/2(Omega) -> Brake Control Unit (BCU)/2(Omega)
  Subsystem3/3(<Acc>) -> Brake Control Unit (BCU)/3(Accel)
  Subsystem2/7(UpReq) -> Transmission Control Unit (TCU)/7(UpReq)
  Subsystem2/8(DnReq) -> Transmission Control Unit (TCU)/8(DownReq)
  Subsystem4/1(Brake) -> [Brake], BusElementOut1/1
  Brake Control Unit (BCU)/1(BrkPrsCmd) -> Subsystem4/1(BrkPrsCmd)
  Brake Control Unit (BCU)/2(ABSFlag) -> Subsystem4/2(ABSFlag)

== system ConfiguredVirtualVehicleModel/Environment ==
  note: GRADE AND GROUND SIGNALS ARE CURRENTLY NOT AFFECTING WHEEL CONTACT. HOWEVER, THEY WILL BE USED IN A FUTURE RELEASE
  note: The Ground Feedback variant subsystem is automatically enabled/disabled according to the 3D Engine settings found in the Reference Generator.
      | Manually overriding this variant may result in initialization errors.
  In Bus Element1 : Inport  PortName=MotoFdbk
  Bus Creator : BusCreator  Inputs=3
  Bus Creator1 : BusCreator  Inputs=5
  Bus Selector : BusSelector  OutputSignals=Whl.Genrl.Frnt.Cp.Disp.z,Whl.Genrl.Rear.Cp.Disp.z,Wheels.FrontTire.Omega,Wheels.RearTire.Omega,Wheels.FrontTire.Alpha,Wheels.RearTire.Alpha
  Bus to Vector : BusToVector
  Bus to Vector1 : BusToVector
  Bus to Vector2 : BusToVector
  Constant : Constant  Value=zeros(1,2)
  Constant1 : Constant  Value=zeros(1,2)
  Constant2 : Constant  Value=EnvWindVelX  SampleTime=0
  Constant4 : Constant  Value=EnvWindVelY  SampleTime=0
  Constant5 : Constant  Value=EnvWindVelZ  SampleTime=0
  EnvAbsPrs_Pa : Constant  Value=EnvAbsPrs  SampleTime=0
  Estimated Grade : Subsystem
  Friction : Subsystem  Variant=on  VariantControlMode=label  VariantControl=Choice  LabelModeActiveChoice=Constant Friction
  Ground Feedback : Subsystem  Variant=on  VariantControlMode=label  LabelModeActiveChoice=0
  Mux : Mux  Inputs=2
  Mux1 : Mux  Inputs=2
  Mux2 : Mux  Inputs=2
  Reshape : Reshape  OutputDimensionality=Row vector (2-D)
  Reshape1 : Reshape  OutputDimensionality=Row vector (2-D)
  Reshape2 : Reshape  OutputDimensionality=Row vector (2-D)
  Signal Specification : SignalSpecification  Unit=K
  Signal Specification1 : SignalSpecification  Unit=Pa
  Signal Specification2 : SignalSpecification  Unit=m/s
  Temp_degK : Constant  Value=EnvAirTemp  SampleTime=0
  Vector Concatenate : Concatenate  NumInputs=3
  Vector Concatenate1 : Concatenate  NumInputs=3  Mode=Multidimensional array
  Env : Outport  VectorParamsAs1DForOutWhenUnconnected=off
  wires:
  Constant5/1 -> Vector Concatenate/3  "Z"
  Signal Specification2/1 -> Bus Creator1/3  "Wind"
  Constant4/1 -> Vector Concatenate/2  "Y"
  Ground Feedback/1(Ground) -> Bus Creator1/5, Estimated Grade/1(Gnd)  "Gnd"
  Bus Creator1/1 -> Env/1
  Signal Specification/1 -> Bus Creator1/1  "Temp"
  Signal Specification1/1 -> Bus Creator1/2  "Baro"
  Friction/1(FricCoeffLambda) -> Ground Feedback/1(Friction)
  Estimated Grade/1(Grade) -> Bus Creator1/4  "Grade"
  In Bus Element1/1 -> Friction/1(MotoFdbk), Bus Selector/1
  Bus Selector/2 -> Mux/2  "<z>"
  Bus Selector/1 -> Mux/1  "<z>"
  Mux/1 -> Bus to Vector/1
  Bus to Vector/1 -> Bus Creator/1  "z"
  Bus Selector/3 -> Mux1/1  "<Omega>"
  Bus Selector/4 -> Mux1/2  "<Omega>"
  Mux1/1 -> Bus to Vector1/1
  Bus to Vector1/1 -> Bus Creator/2  "Omega"
  Bus Selector/5 -> Mux2/1  "<Alpha>"
  Bus Selector/6 -> Mux2/2  "<Alpha>"
  Mux2/1 -> Bus to Vector2/1
  Constant/1 -> Reshape/1
  Constant1/1 -> Reshape1/1
  Bus to Vector2/1 -> Reshape2/1
  Reshape/1 -> Vector Concatenate1/1
  Reshape1/1 -> Vector Concatenate1/2
  Reshape2/1 -> Vector Concatenate1/3
  Vector Concatenate1/1 -> Bus Creator/3  "WhlAng"
  Bus Creator/1 -> Ground Feedback/2(WheelFdbk)  "WheelFdbk"
  Constant2/1 -> Vector Concatenate/1  "X"
  Temp_degK/1 -> Signal Specification/1
  EnvAbsPrs_Pa/1 -> Signal Specification1/1
  Vector Concatenate/1 -> Signal Specification2/1

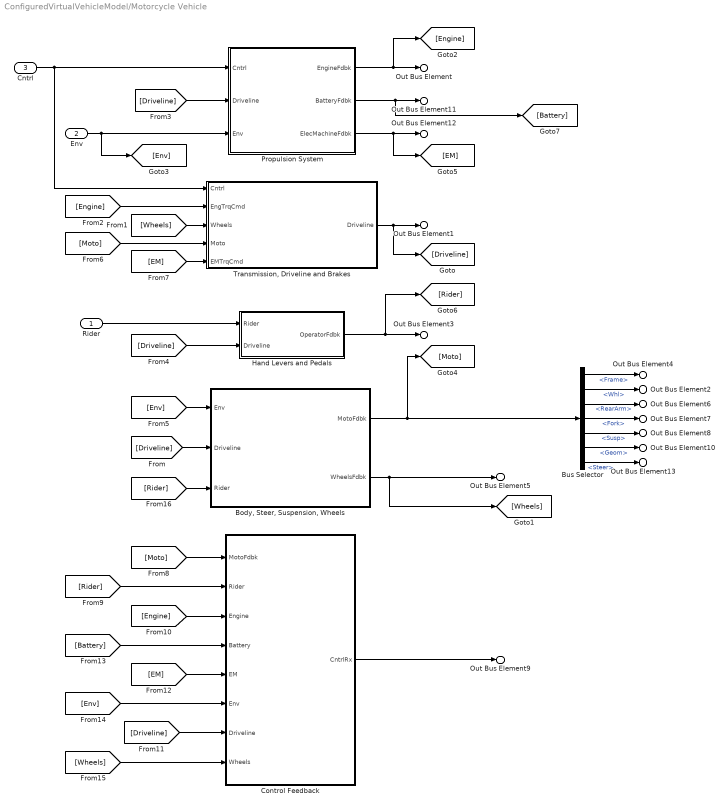
== system ConfiguredVirtualVehicleModel/Motorcycle Vehicle ==
  Rider : Inport
  Env : Inport  Port=2
  Cntrl : Inport  Port=3
  "Body, Steer, Suspension, Wheels" : Subsystem
      mask Display: image('$imagefile'); % Use "Edit Image" on toolstrip to change.
  Bus Selector : BusSelector  OutputSignals=Frame,Whl,RearArm,Fork,Susp,Geom,Steer
  Control Feedback : Subsystem
  Hand Levers and Pedals : Subsystem
  Propulsion System : Subsystem
      mask Display: image('$imagefile'); % Use "Edit Image" on toolstrip to change.
  "Transmission, Driveline and Brakes" : Subsystem
      mask Display: image('$imagefile'); % Use "Edit Image" on toolstrip to change.
  Out Bus Element : Outport  PortName=MotoFdbk  Element=Engine
  Out Bus Element3 : Outport  PortName=MotoFdbk  Element=Rider
  Out Bus Element4 : Outport  PortName=MotoFdbk  Element=Body
  Out Bus Element5 : Outport  PortName=MotoFdbk  Element=Wheels
  Out Bus Element1 : Outport  PortName=MotoFdbk  Element=Driveline
  Out Bus Element2 : Outport  PortName=MotoFdbk  Element=Whl
  Out Bus Element6 : Outport  PortName=MotoFdbk  Element=RearArm
  Out Bus Element7 : Outport  PortName=MotoFdbk  Element=Fork
  Out Bus Element8 : Outport  PortName=MotoFdbk  Element=Susp
  Out Bus Element10 : Outport  PortName=MotoFdbk  Element=Geom
  Out Bus Element11 : Outport  PortName=MotoFdbk  Element=Battery
  Out Bus Element12 : Outport  PortName=MotoFdbk  Element=ElecMachine
  Out Bus Element13 : Outport  PortName=MotoFdbk  Element=Steer
  Out Bus Element9 : Outport  Port=2  PortName=CntrlFdbk
  wires:
  Bus Selector/1 -> Out Bus Element4/1  "<Frame>"
  Bus Selector/2 -> Out Bus Element2/1  "<Whl>"
  Bus Selector/3 -> Out Bus Element6/1  "<RearArm>"
  Bus Selector/4 -> Out Bus Element7/1  "<Fork>"
  Bus Selector/5 -> Out Bus Element8/1  "<Susp>"
  Bus Selector/6 -> Out Bus Element10/1  "<Geom>"
  Propulsion System/1(EngineFdbk) -> [Engine], Out Bus Element/1
  [Driveline] -> Propulsion System/2(Driveline)
  "Transmission, Driveline and Brakes"/1(Driveline) -> [Driveline], Out Bus Element1/1
  [Engine] -> "Transmission, Driveline and Brakes"/2(EngTrqCmd)
  [Wheels] -> "Transmission, Driveline and Brakes"/3(Wheels)
  [Moto] -> "Transmission, Driveline and Brakes"/4(Moto)
  Propulsion System/2(BatteryFdbk) -> [Battery], Out Bus Element11/1
  Propulsion System/3(ElecMachineFdbk) -> Out Bus Element12/1, [EM]
  Rider/1 -> Hand Levers and Pedals/1(Rider)
  [Driveline] -> Hand Levers and Pedals/2(Driveline)
  Hand Levers and Pedals/1(OperatorFdbk) -> [Rider], Out Bus Element3/1
  "Body, Steer, Suspension, Wheels"/1(MotoFdbk) -> Bus Selector/1, [Moto]
  "Body, Steer, Suspension, Wheels"/2(WheelsFdbk) -> [Wheels], Out Bus Element5/1
  [Driveline] -> "Body, Steer, Suspension, Wheels"/2(Driveline)
  Env/1 -> [Env], Propulsion System/3(Env)
  [Env] -> "Body, Steer, Suspension, Wheels"/1(Env)
  [EM] -> "Transmission, Driveline and Brakes"/5(EMTrqCmd)
  Cntrl/1 -> "Transmission, Driveline and Brakes"/1(Cntrl), Propulsion System/1(Cntrl)
  Control Feedback/1(CntrlRx) -> Out Bus Element9/1
  [Moto] -> Control Feedback/1(MotoFdbk)
  [Rider] -> Control Feedback/2(Rider)
  [Engine] -> Control Feedback/3(Engine)
  [EM] -> Control Feedback/5(EM)
  [Battery] -> Control Feedback/4(Battery)
  [Driveline] -> Control Feedback/7(Driveline)
  [Env] -> Control Feedback/6(Env)
  [Wheels] -> Control Feedback/8(Wheels)
  [Rider] -> "Body, Steer, Suspension, Wheels"/3(Rider)
  Bus Selector/7 -> Out Bus Element13/1  "<Steer>"

== system ConfiguredVirtualVehicleModel/Reference Generator for Motorcycle ==
  "MotoFdbk " : Inport
  3D Engine : Subsystem  Variant=on  VariantControlMode=label  LabelModeActiveChoice=Disabled  mask(3D Engine){engine3D=Disabled, SceneDesc=Open surface, dt3D=dt3D, defaultPos=Recommended for scene, X_o=X_o, Y_o=Y_o, Z_o=Z_o, phi_o=phi_o, theta_o=theta_o, psi_o=psi_o}
      mask prompts: engine3D "3D Engine"; SceneDesc "shared_sim3dblks:sim3dblkConfig:SceneDesc"; dt3D "Engine frame rate, dt3D [s]:"; X_o "Initial longitudinal position, X_o [m]:"; Y_o "Initial lateral position, Y_o [m]:"; Z_o "Initial vertical position, Z_o [m]:"; phi_o "Initial roll angle, phi_o [rad]:"; theta_o "Initial pitch angle, theta_o [rad]:"; psi_o "Initial yaw angle, psi_o [rad]:"
      mask help: This subsystem contains the interface blocks which permit the display of the vehicle in the 3D virtual environment. Enable it to view the simulation progress, disable it to inhibit the display.
      settings: AttributesFormatString=|
      | %<SceneDesc>
      | %<engine3D>
      mask Help: eval('vdynblkshelp(''vdynblks3dengine'')');
      mask TypeOptions engine3D: vdynblks:vehdynRefApp3DEng:blkRdBt_engine3D_c2 | vdynblks:vehdynRefApp3DEng:blkRdBt_engine3D_c1
      mask Callback engine3D:
      | sim3denabled=get_param(gcb,'engine3D');
      | %set_param(gcb,'OverrideUsingVariant',sim3denabled);
      | GrndFdbkPath = [bdroot(gcb) '/Environment/Ground Feedback'];
      | switch sim3denabled
      |     case 'Disabled'
      |         try
      |             set_param(GrndFdbkPath,'LabelModeActiveChoice','0');
      |             set_param([bdroot(gcb) '/Reference Generator for Motorcycle/Reference Generator/Double Lane Change/Double Lane Change'],'use3DCones','off');
      |             set_param([bdroot(gcb) '/Reference Generator for Motorcycle/Reference Generator/Constant Radius'],'use3DCones','off');
      |         catch
      |             disp('Warning: Ground feedback source subsystem was not found. Ground feedback source remains unchanged.');
      |         end
      |     case 'Enabled'
      |         try
      |             set_param(GrndFdbkPath,'LabelModeActiveChoice','1');
      |             set_param([bdroot(gcb) '/Reference Generator for Motorcycle/Reference Generator/Double Lane Change/Double Lane Change'],'use3DCones','on');
      |             set_param([bdroot(gcb) '/Reference Generator for Motorcycle/Reference Generator/Constant Radius'],'use3DCones','on');
      |         catch
      |             disp('Warning: Ground feedback source subsystem was not found. Ground feedback source remains unchanged.');
      |         end
      |     otherwise
      | end
      mask TypeOptions SceneDesc: 3D Engine/Simulation 3D Scene Configuration/SceneDesc
      mask Callback SceneDesc: [~] = vdynblks3Dsceneconfig(gcb);
      mask TypeOptions defaultPos: vdynblks:vehdynRefApp3DEng:blkRdBt_defaultPos_c1 | vdynblks:vehdynRefApp3DEng:blkRdBt_defaultPos_c2
      mask DialogControl engineConfig Prompt: 3D Engine Settings
      mask DialogControl SceneDesc Prompt: Scene name:
      mask DialogControl posSetup Prompt: Initial vehicle position
      mask DialogControl posSetupDesc Prompt: To use these initial vehicle positions, first Apply the initial values and then click Update the model workspaces with the initial values.
      mask DialogControl setModelPos Prompt: Update model workspaces with initial values
      mask DialogControl setModelPos Callback: [~] = vdynblksmdlWSconfig(gcb);
      mask Display: disp('3D Engine')
  Reference Generator : Subsystem  Variant=on  VariantControlMode=label  VariantControl=Variant1  LabelModeActiveChoice=Drive Cycle
  Reference Router : Subsystem  Variant=on  VariantControlMode=label  LabelModeActiveChoice=Maneuver Tracking
  " Vis" : Outport  VectorParamsAs1DForOutWhenUnconnected=off
  " Ref" : Outport  Port=2  VectorParamsAs1DForOutWhenUnconnected=off
  " Fdbk" : Outport  Port=3  VectorParamsAs1DForOutWhenUnconnected=off
  wires:
  "MotoFdbk "/1 -> Reference Generator/1("MotoFdbk "), 3D Engine/1(MotoFdbk)
  Reference Generator/1(" Vis") -> Reference Router/1(VisIn)
  Reference Generator/2(" Ref") -> Reference Router/2(RefIn)
  Reference Generator/3(" Fdbk") -> Reference Router/3(FdbkIn)
  Reference Router/1(Vis) -> " Vis"/1
  Reference Router/2(Ref) -> " Ref"/1
  Reference Router/3(Fdbk) -> " Fdbk"/1

== system ConfiguredVirtualVehicleModel/Rider Commands ==
  MotoRef : Inport
  MotoFdbk : Inport  Port=2
  Env : Inport  Port=3
  GearGround : Ground
  Rider Commands : Subsystem  Variant=on  VariantControl=Variant1
  Torque Control : Subsystem  Variant=on
  Rider : Outport  VectorParamsAs1DForOutWhenUnconnected=off
  wires:
  MotoRef/1 -> Torque Control/1(MotoRef), Rider Commands/1(MotoRef)
  MotoFdbk/1 -> Torque Control/2(MotoFdbk), Rider Commands/2(MotoFdbk)
  Rider Commands/1(" Rider") -> Torque Control/3(RiderInput)
  Env/1 -> Rider Commands/3(Env)
  Torque Control/1(Rider) -> Rider/1
  GearGround/1 -> Rider Commands/4(GearCmd)
